simulink model "Proj2_P4"  (Simulink 8.6)
settings: Solver=ode45  StartTime=0.0  StopTime=10  MaxStep=0.001  RelTol=1e-3
values from neighbouring files (symbols this model uses):
  fl_rd_0 = fl_rd_rated    [Proj2_IM_IC_rated.m]    (also in Proj2_P1_calc.m = eps)
  fl_rd_0_est2 = fl_rd_rated_est2    [Proj2_P4_S2.m]    (also in Proj2_P4_calc2.m = fl_rd_0; Proj2_P4_calc3.m = fl_rd_0)
  fl_rd_0_est3 = fl_rd_rated    [Proj2_P4_S3.m]    (also in Proj2_P4_calc2.m = fl_rd_0; Proj2_P4_calc3.m = fl_rd_0)
  fl_sd_0 = fl_sd_rated    [Proj2_IM_IC_rated.m]    (also in Proj2_P1_calc.m = 0)
  fl_sq_0 = fl_sq_rated    [Proj2_IM_IC_rated.m]    (also in Proj2_P1_calc.m = 0)
  Isd_rated = real(Is_rated)    [Proj2_IM_IC_rated.m]
  Isd_rated_est2 = real(Is_rated_est2)    [Proj2_P4_S2.m]    (also in Proj2_P4_calc2.m = Isd_rated)
  Isd_rated_est3 = real(Is_rated_est3)    [Proj2_P4_S3.m]    (also in Proj2_P4_calc2.m = Isd_rated)
  Isq_0 = Isq_rated    [Proj2_IM_IC_rated.m]
  Isq_0_est2 = Isq_rated_est2    [Proj2_P4_S2.m]    (also in Proj2_P4_calc2.m = Isq_0; Proj2_P4_calc3.m = Isq_0)
  Isq_0_est3 = Isq_rated_est3    [Proj2_P4_S3.m]    (also in Proj2_P4_calc2.m = Isq_0; Proj2_P4_calc3.m = Isq_0)
  J_eq = 75    [Proj2_IM_parameters.m]
  Ki_i = w_c_i*sqrt(R_s^2+(w_c_i*L_s*sigma)^2) / sqrt(1+wc_Kp_by_Ki_for_i^2)    [Proj2_IM_IC_rated.m]
  Ki_i_est3 = w_c_i*sqrt(R_s^2+(w_c_i*L_s*sigma_est3)^2) / sqrt(1+wc_Kp_by_Ki_for_i_est3^2)    [Proj2_P4_S3.m]    (also in Proj2_P4_calc2.m = Ki_i)
  Ki_s = w_c_s^2*J_eq/(k*sqrt(1+tan(PM_s)^2))    [Proj2_IM_IC_rated.m]
  Ki_s_est2 = w_c_s^2*J_eq/(k_est2*sqrt(1+tan(PM_s)^2))    [Proj2_P4_S2.m]    (also in Proj2_P4_calc2.m = Ki_s)
  Ki_s_est3 = w_c_s^2*J_eq/(k_est3*sqrt(1+tan(PM_s)^2))    [Proj2_P4_S3.m]    (also in Proj2_P4_calc2.m = Ki_s)
  Kp_i = Ki_i * wc_Kp_by_Ki_for_i / w_c_i    [Proj2_IM_IC_rated.m]
  Kp_i_est3 = Ki_i_est3 * wc_Kp_by_Ki_for_i_est3 / w_c_i    [Proj2_P4_S3.m]    (also in Proj2_P4_calc2.m = Kp_i)
  Kp_s = Ki_s * wc_Kp_by_Ki_for_s / w_c_s    [Proj2_IM_IC_rated.m]
  Kp_s_est2 = Ki_s_est2 * wc_Kp_by_Ki_for_s / w_c_s    [Proj2_P4_S2.m]    (also in Proj2_P4_calc2.m = Kp_s)
  Kp_s_est3 = Ki_s_est3 * wc_Kp_by_Ki_for_s / w_c_s    [Proj2_P4_S3.m]    (also in Proj2_P4_calc2.m = Kp_s)
  L_m = X_m /w_syn    (= 0.00152788745368)    [Proj2_IM_parameters.m]
  L_r = L_lr+L_m    (= 0.00161011750761)    [Proj2_IM_parameters.m]
  L_r_est3 = L_lr_est3 + L_m    [Proj2_P4_S3.m]
  L_s = L_ls+L_m    (= 0.00161807525477)    [Proj2_IM_parameters.m]
  p = 6    [Proj2_IM_parameters.m]
  R_s = 1.4*10^-3    (= 0.0014)    [Proj2_IM_parameters.m]
  sigma = 1-L_m^2/(L_s*L_r)    (= 0.103961973695)    [Proj2_IM_parameters.m]
  sigma_est3 = 1-L_m^2/(L_s*L_r_est3)    [Proj2_P4_S3.m]
  T_L_rated = T_em_rated    [Proj2_IM_parameters.m]
  tau_r = L_r/R_r    (= 1.62474016914)    [Proj2_IM_parameters.m]
  tau_r_est2 = L_r/R_r_est2    [Proj2_P4_S2.m]
  tau_r_est3 = L_r_est3/R_r    [Proj2_P4_S3.m]
  theta_da_0 = theta_fl_rated_a    [Proj2_IM_IC_rated.m]    (also in Proj2_P1_calc.m = 0)
  theta_dA_0 = theta_fl_rated_a    [Proj2_IM_IC_rated.m]    (also in Proj2_P1_calc.m = 0)
  theta_da_0_est2 = theta_fl_rated_a_est2    [Proj2_P4_S2.m]    (also in Proj2_P4_calc2.m = theta_da_0; Proj2_P4_calc3.m = theta_da_0)
  theta_da_0_est3 = theta_fl_rated_a_est3    [Proj2_P4_S3.m]    (also in Proj2_P4_calc2.m = theta_da_0; Proj2_P4_calc3.m = theta_da_0)
  Vsd_prime_0 = Vsd_0 - L_m/L_r*d_fl_rd_0_by_dt + w_syn*sigma*L_s*Isq_0    [Proj2_IM_IC_rated.m]
  Vsd_prime_0_est2 = Vsd_0 - L_m/L_r*d_fl_rd_0_by_dt_est2 + w_syn*sigma*L_s*Isq_0_est2    [Proj2_P4_S2.m]    (also in Proj2_P4_calc2.m = Vsd_prime_0; Proj2_P4_calc3.m = Vsd_prime_0)
  Vsd_prime_0_est3 = Vsd_0 - L_m/L_r_est3*d_fl_rd_0_by_dt_est3 + w_syn*sigma_est3*L_s*Isq_0_est3    [Proj2_P4_S3.m]    (also in Proj2_P4_calc2.m = Vsd_prime_0; Proj2_P4_calc3.m = Vsd_prime_0)
  Vsq_prime_0 = Vsq_0 - w_syn*(L_m/L_r)*fl_rd_0 - w_syn*sigma*L_s*Isd_0    [Proj2_IM_IC_rated.m]
  Vsq_prime_0_est2 = Vsq_0 - w_syn*(L_m/L_r)*fl_rd_0_est2 - w_syn*sigma*L_s*Isd_0_est2    [Proj2_P4_S2.m]    (also in Proj2_P4_calc2.m = Vsq_prime_0; Proj2_P4_calc3.m = Vsq_prime_0)
  Vsq_prime_0_est3 = Vsq_0 - w_syn*(L_m/L_r_est3)*fl_rd_0_est3 - w_syn*sigma_est3*L_s*Isd_0_est3    [Proj2_P4_S3.m]    (also in Proj2_P4_calc2.m = Vsq_prime_0; Proj2_P4_calc3.m = Vsq_prime_0)
  w_mech_0 = w_mech_rated    [Proj2_IM_IC_rated.m]    (also in Proj2_P1_calc.m = 0)
  w_mech_rated = (1-s)*w_syn/(p/2)    (= 124.407069082)    [Proj2_IM_parameters.m]
(part 2 of 2)

== system Proj2_P4/Actual Motor dq Model Modified from EX5_3  /dq --> abc Eq. 2.10 ==
  d : Inport
  q : Inport  Port=2
  theta_da : Inport  Port=3
  Mux1 : Mux  Inputs=3
  ia Eq. 3-18 : Fcn  Expr=sqrt(2/3)*(cos(u(3))*u(1)-sin(u(3))*u(2))
  ib Eq. 3-18 : Fcn  Expr=sqrt(2/3)*(cos(u(3)+4*pi/3)*u(1)-sin(u(3)+4*pi/3)*u(2))
  ic Eq. 3-18 : Fcn  Expr=sqrt(2/3)*(cos(u(3)+2*pi/3)*u(1)-sin(u(3)+2*pi/3)*u(2))
  ia : Outport
  ib : Outport  Port=2
  ic : Outport  Port=3
  wires:
  ic Eq. 3-18/1 -> ic/1
  Mux1/1 -> ic Eq. 3-18/1, ib Eq. 3-18/1, ia Eq. 3-18/1
  ia Eq. 3-18/1 -> ia/1
  ib Eq. 3-18/1 -> ib/1
  d/1 -> Mux1/1
  q/1 -> Mux1/2
  theta_da/1 -> Mux1/3

== system Proj2_P4/Actual Motor dq Model Modified from EX5_3  /dq --> abc Eq. 2.16  ==
  d : Inport
  q : Inport  Port=2
  theta_dA : Inport  Port=3
  Mux1 : Mux  Inputs=3
  ia Eq. 3-18 : Fcn  Expr=sqrt(2/3)*(cos(u(3))*u(1)-sin(u(3))*u(2))
  ib Eq. 3-18 : Fcn  Expr=sqrt(2/3)*(cos(u(3)+4*pi/3)*u(1)-sin(u(3)+4*pi/3)*u(2))
  ic Eq. 3-18 : Fcn  Expr=sqrt(2/3)*(cos(u(3)+2*pi/3)*u(1)-sin(u(3)+2*pi/3)*u(2))
  i_A : Outport
  i_B : Outport  Port=2
  i_C : Outport  Port=3
  wires:
  ic Eq. 3-18/1 -> i_C/1
  Mux1/1 -> ic Eq. 3-18/1, ib Eq. 3-18/1, ia Eq. 3-18/1
  ib Eq. 3-18/1 -> i_B/1
  d/1 -> Mux1/1
  q/1 -> Mux1/2
  theta_dA/1 -> Mux1/3
  ia Eq. 3-18/1 -> i_A/1

== system Proj2_P4/Actual Motor dq Model Modified from EX5_3  /stator_flux Eq. 2.28 ==
  vs_dq : Inport
  is_dq : Inport  Port=2
  w_d : Inport  Port=3
  Gain : Gain  Gain=R_s  SaturateOnIntegerOverflow=on  OutDataTypeStr=Inherit: Same as input  ParamDataTypeStr=Inherit: Same as input
  Integrator1 : Integrator  InitialCondition=[fl_sd_0; fl_sq_0]
  "Matrix [0 -1  1 0] " : Gain  Gain=[0 -1; 1 0]  Multiplication=Matrix(K*u)  SaturateOnIntegerOverflow=on  OutDataTypeStr=Inherit: Same as input  ParamDataTypeStr=Inherit: Same as input
  Product : Product  SaturateOnIntegerOverflow=on  RndMeth=Zero  InputSameDT=on  OutDataTypeStr=Inherit: Same as first input
  Sum : Sum  Inputs=-+-  SaturateOnIntegerOverflow=on  InputSameDT=on  OutDataTypeStr=Inherit: Same as first input
  fl_s_dq : Outport
  wires:
  Sum/1 -> Integrator1/1
  Integrator1/1 -> "Matrix [0 -1  1 0] "/1, fl_s_dq/1
  "Matrix [0 -1  1 0] "/1 -> Product/2
  Product/1 -> Sum/1
  w_d/1 -> Product/1
  vs_dq/1 -> Sum/2
  is_dq/1 -> Gain/1
  Gain/1 -> Sum/3

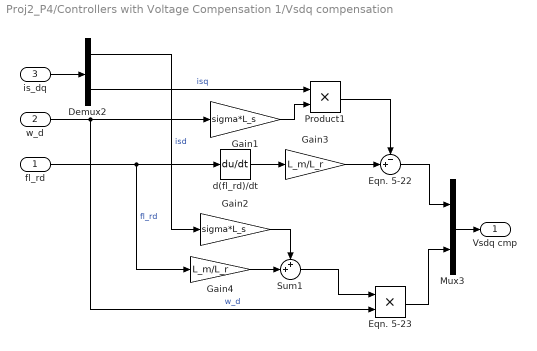
== system Proj2_P4/Controllers with Voltage Compensation 1/Vsdq compensation ==
  fl_rd : Inport
  w_d : Inport  Port=2
  is_dq : Inport  Port=3
  Demux2 : Demux  Outputs=2
  Eqn. 5-22 : Sum  Inputs=-+|  SaturateOnIntegerOverflow=on  InputSameDT=on  OutDataTypeStr=Inherit: Same as first input
  Eqn. 5-23 : Product  RndMeth=Zero
  Gain1 : Gain  Gain=sigma*L_s  SaturateOnIntegerOverflow=on  OutDataTypeStr=Inherit: Same as input  ParamDataTypeStr=Inherit: Same as input
  Gain2 : Gain  Gain=sigma*L_s  SaturateOnIntegerOverflow=on  OutDataTypeStr=Inherit: Same as input  ParamDataTypeStr=Inherit: Same as input
  Gain3 : Gain  Gain=L_m/L_r  SaturateOnIntegerOverflow=on  OutDataTypeStr=Inherit: Same as input  ParamDataTypeStr=Inherit: Same as input
  Gain4 : Gain  Gain=L_m/L_r  SaturateOnIntegerOverflow=on  OutDataTypeStr=Inherit: Same as input  ParamDataTypeStr=Inherit: Same as input
  Mux3 : Mux  Inputs=2
  Product1 : Product  RndMeth=Zero
  Sum1 : Sum  Inputs=++|  SaturateOnIntegerOverflow=on  InputSameDT=on  OutDataTypeStr=Inherit: Same as first input
  d(fl_rd)/dt : Derivative
  Vsdq cmp : Outport
  wires:
  fl_rd/1 -> d(fl_rd)/dt/1, Gain4/1  "fl_rd"
  d(fl_rd)/dt/1 -> Gain3/1
  Gain3/1 -> Eqn. 5-22/2
  w_d/1 -> Gain1/1, Eqn. 5-23/2  "w_d"
  Gain1/1 -> Product1/2
  Product1/1 -> Eqn. 5-22/1
  Eqn. 5-22/1 -> Mux3/1
  is_dq/1 -> Demux2/1
  Demux2/2 -> Product1/1  "isq"
  Gain4/1 -> Sum1/2
  Gain2/1 -> Sum1/1
  Sum1/1 -> Eqn. 5-23/1
  Eqn. 5-23/1 -> Mux3/2
  Demux2/1 -> Gain2/1  "isd"
  Mux3/1 -> Vsdq cmp/1

== system Proj2_P4/Controllers with Voltage Compensation 1/abc --> dq ==
  a : Inport
  b : Inport  Port=2
  c : Inport  Port=3
  theta_da_est : Inport  Port=4
  Mux1 : Mux
  isd Eq. 3-12 : Fcn  Expr=sqrt(2/3)*(cos(u(4))*u(1)+cos(u(4)-2*pi/3)*u(2)+cos(u(4)-4*pi/3)*u(3))
  isq Eq. 3-12 : Fcn  Expr=-sqrt(2/3)*(sin(u(4))*u(1)+sin(u(4)-2*pi/3)*u(2)+sin(u(4)-4*pi/3)*u(3))
  is_d : Outport
  is_q : Outport  Port=2
  wires:
  theta_da_est/1 -> Mux1/4
  c/1 -> Mux1/3
  b/1 -> Mux1/2
  a/1 -> Mux1/1
  isq Eq. 3-12/1 -> is_q/1
  isd Eq. 3-12/1 -> is_d/1
  Mux1/1 -> isq Eq. 3-12/1, isd Eq. 3-12/1

== system Proj2_P4/Controllers with Voltage Compensation 1/dq --> abc  ==
  d : Inport
  q : Inport  Port=2
  theta_da_est : Inport  Port=3
  Mux1 : Mux  Inputs=3
  ia Eq. 3-18 : Fcn  Expr=sqrt(2/3)*(cos(u(3))*u(1)-sin(u(3))*u(2))
  ib Eq. 3-18 : Fcn  Expr=sqrt(2/3)*(cos(u(3)+4*pi/3)*u(1)-sin(u(3)+4*pi/3)*u(2))
  ic Eq. 3-18 : Fcn  Expr=sqrt(2/3)*(cos(u(3)+2*pi/3)*u(1)-sin(u(3)+2*pi/3)*u(2))
  Va : Outport
  Vb : Outport  Port=2
  Vc : Outport  Port=3
  wires:
  ic Eq. 3-18/1 -> Vc/1
  Mux1/1 -> ic Eq. 3-18/1, ib Eq. 3-18/1, ia Eq. 3-18/1
  ib Eq. 3-18/1 -> Vb/1
  d/1 -> Mux1/1
  q/1 -> Mux1/2
  theta_da_est/1 -> Mux1/3
  ia Eq. 3-18/1 -> Va/1

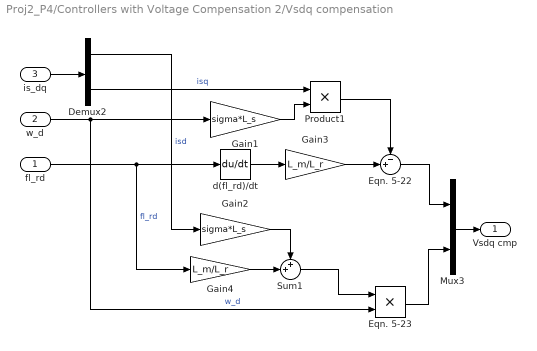
== system Proj2_P4/Controllers with Voltage Compensation 2/Vsdq compensation ==
  fl_rd : Inport
  w_d : Inport  Port=2
  is_dq : Inport  Port=3
  Demux2 : Demux  Outputs=2
  Eqn. 5-22 : Sum  Inputs=-+|  SaturateOnIntegerOverflow=on  InputSameDT=on  OutDataTypeStr=Inherit: Same as first input
  Eqn. 5-23 : Product  RndMeth=Zero
  Gain1 : Gain  Gain=sigma*L_s  SaturateOnIntegerOverflow=on  OutDataTypeStr=Inherit: Same as input  ParamDataTypeStr=Inherit: Same as input
  Gain2 : Gain  Gain=sigma*L_s  SaturateOnIntegerOverflow=on  OutDataTypeStr=Inherit: Same as input  ParamDataTypeStr=Inherit: Same as input
  Gain3 : Gain  Gain=L_m/L_r  SaturateOnIntegerOverflow=on  OutDataTypeStr=Inherit: Same as input  ParamDataTypeStr=Inherit: Same as input
  Gain4 : Gain  Gain=L_m/L_r  SaturateOnIntegerOverflow=on  OutDataTypeStr=Inherit: Same as input  ParamDataTypeStr=Inherit: Same as input
  Mux3 : Mux  Inputs=2
  Product1 : Product  RndMeth=Zero
  Sum1 : Sum  Inputs=++|  SaturateOnIntegerOverflow=on  InputSameDT=on  OutDataTypeStr=Inherit: Same as first input
  d(fl_rd)/dt : Derivative
  Vsdq cmp : Outport
  wires:
  fl_rd/1 -> d(fl_rd)/dt/1, Gain4/1  "fl_rd"
  d(fl_rd)/dt/1 -> Gain3/1
  Gain3/1 -> Eqn. 5-22/2
  w_d/1 -> Gain1/1, Eqn. 5-23/2  "w_d"
  Gain1/1 -> Product1/2
  Product1/1 -> Eqn. 5-22/1
  Eqn. 5-22/1 -> Mux3/1
  is_dq/1 -> Demux2/1
  Demux2/2 -> Product1/1  "isq"
  Gain4/1 -> Sum1/2
  Gain2/1 -> Sum1/1
  Sum1/1 -> Eqn. 5-23/1
  Eqn. 5-23/1 -> Mux3/2
  Demux2/1 -> Gain2/1  "isd"
  Mux3/1 -> Vsdq cmp/1

== system Proj2_P4/Controllers with Voltage Compensation 2/abc --> dq  ==
  a : Inport
  b : Inport  Port=2
  c : Inport  Port=3
  theta_da_est : Inport  Port=4
  Mux1 : Mux
  isd Eq. 3-12 : Fcn  Expr=sqrt(2/3)*(cos(u(4))*u(1)+cos(u(4)-2*pi/3)*u(2)+cos(u(4)-4*pi/3)*u(3))
  isq Eq. 3-12 : Fcn  Expr=-sqrt(2/3)*(sin(u(4))*u(1)+sin(u(4)-2*pi/3)*u(2)+sin(u(4)-4*pi/3)*u(3))
  is_d : Outport
  is_q : Outport  Port=2
  wires:
  theta_da_est/1 -> Mux1/4
  c/1 -> Mux1/3
  b/1 -> Mux1/2
  a/1 -> Mux1/1
  isq Eq. 3-12/1 -> is_q/1
  isd Eq. 3-12/1 -> is_d/1
  Mux1/1 -> isq Eq. 3-12/1, isd Eq. 3-12/1

== system Proj2_P4/Controllers with Voltage Compensation 2/dq --> abc  ==
  d : Inport
  q : Inport  Port=2
  theta_da_est : Inport  Port=3
  Mux1 : Mux  Inputs=3
  ia Eq. 3-18 : Fcn  Expr=sqrt(2/3)*(cos(u(3))*u(1)-sin(u(3))*u(2))
  ib Eq. 3-18 : Fcn  Expr=sqrt(2/3)*(cos(u(3)+4*pi/3)*u(1)-sin(u(3)+4*pi/3)*u(2))
  ic Eq. 3-18 : Fcn  Expr=sqrt(2/3)*(cos(u(3)+2*pi/3)*u(1)-sin(u(3)+2*pi/3)*u(2))
  Va : Outport
  Vb : Outport  Port=2
  Vc : Outport  Port=3
  wires:
  ic Eq. 3-18/1 -> Vc/1
  Mux1/1 -> ic Eq. 3-18/1, ib Eq. 3-18/1, ia Eq. 3-18/1
  ib Eq. 3-18/1 -> Vb/1
  d/1 -> Mux1/1
  q/1 -> Mux1/2
  theta_da_est/1 -> Mux1/3
  ia Eq. 3-18/1 -> Va/1

== system Proj2_P4/Controllers with Voltage Compensation 3/Vsdq compensation ==
  fl_rd : Inport
  w_d : Inport  Port=2
  is_dq : Inport  Port=3
  Demux2 : Demux  Outputs=2
  Eqn. 5-22 : Sum  Inputs=-+|  SaturateOnIntegerOverflow=on  InputSameDT=on  OutDataTypeStr=Inherit: Same as first input
  Eqn. 5-23 : Product  RndMeth=Zero
  Gain1 : Gain  Gain=sigma_est3*L_s  SaturateOnIntegerOverflow=on  OutDataTypeStr=Inherit: Same as input  ParamDataTypeStr=Inherit: Same as input
  Gain2 : Gain  Gain=sigma_est3*L_s  SaturateOnIntegerOverflow=on  OutDataTypeStr=Inherit: Same as input  ParamDataTypeStr=Inherit: Same as input
  Gain3 : Gain  Gain=L_m/L_r_est3  SaturateOnIntegerOverflow=on  OutDataTypeStr=Inherit: Same as input  ParamDataTypeStr=Inherit: Same as input
  Gain4 : Gain  Gain=L_m/L_r_est3  SaturateOnIntegerOverflow=on  OutDataTypeStr=Inherit: Same as input  ParamDataTypeStr=Inherit: Same as input
  Mux3 : Mux  Inputs=2
  Product1 : Product  RndMeth=Zero
  Sum1 : Sum  Inputs=++|  SaturateOnIntegerOverflow=on  InputSameDT=on  OutDataTypeStr=Inherit: Same as first input
  d(fl_rd)/dt : Derivative
  Vsdq cmp : Outport
  wires:
  fl_rd/1 -> d(fl_rd)/dt/1, Gain4/1  "fl_rd"
  d(fl_rd)/dt/1 -> Gain3/1
  Gain3/1 -> Eqn. 5-22/2
  w_d/1 -> Gain1/1, Eqn. 5-23/2  "w_d"
  Gain1/1 -> Product1/2
  Product1/1 -> Eqn. 5-22/1
  Eqn. 5-22/1 -> Mux3/1
  is_dq/1 -> Demux2/1
  Demux2/2 -> Product1/1  "isq"
  Gain4/1 -> Sum1/2
  Gain2/1 -> Sum1/1
  Sum1/1 -> Eqn. 5-23/1
  Eqn. 5-23/1 -> Mux3/2
  Demux2/1 -> Gain2/1  "isd"
  Mux3/1 -> Vsdq cmp/1

== system Proj2_P4/Controllers with Voltage Compensation 3/abc --> dq  ==
  a : Inport
  b : Inport  Port=2
  c : Inport  Port=3
  theta_da_est : Inport  Port=4
  Mux1 : Mux
  isd Eq. 3-12 : Fcn  Expr=sqrt(2/3)*(cos(u(4))*u(1)+cos(u(4)-2*pi/3)*u(2)+cos(u(4)-4*pi/3)*u(3))
  isq Eq. 3-12 : Fcn  Expr=-sqrt(2/3)*(sin(u(4))*u(1)+sin(u(4)-2*pi/3)*u(2)+sin(u(4)-4*pi/3)*u(3))
  is_d : Outport
  is_q : Outport  Port=2
  wires:
  theta_da_est/1 -> Mux1/4
  c/1 -> Mux1/3
  b/1 -> Mux1/2
  a/1 -> Mux1/1
  isq Eq. 3-12/1 -> is_q/1
  isd Eq. 3-12/1 -> is_d/1
  Mux1/1 -> isq Eq. 3-12/1, isd Eq. 3-12/1

== system Proj2_P4/Controllers with Voltage Compensation 3/dq --> abc  ==
  d : Inport
  q : Inport  Port=2
  theta_da_est : Inport  Port=3
  Mux1 : Mux  Inputs=3
  ia Eq. 3-18 : Fcn  Expr=sqrt(2/3)*(cos(u(3))*u(1)-sin(u(3))*u(2))
  ib Eq. 3-18 : Fcn  Expr=sqrt(2/3)*(cos(u(3)+4*pi/3)*u(1)-sin(u(3)+4*pi/3)*u(2))
  ic Eq. 3-18 : Fcn  Expr=sqrt(2/3)*(cos(u(3)+2*pi/3)*u(1)-sin(u(3)+2*pi/3)*u(2))
  Va : Outport
  Vb : Outport  Port=2
  Vc : Outport  Port=3
  wires:
  ic Eq. 3-18/1 -> Vc/1
  Mux1/1 -> ic Eq. 3-18/1, ib Eq. 3-18/1, ia Eq. 3-18/1
  ib Eq. 3-18/1 -> Vb/1
  d/1 -> Mux1/1
  q/1 -> Mux1/2
  theta_da_est/1 -> Mux1/3
  ia Eq. 3-18/1 -> Va/1

== system Proj2_P4/Estimated Motor Model/abc --> dq Eq. 3-12 ==
  a : Inport
  b : Inport  Port=2
  c : Inport  Port=3
  theta_da_est : Inport  Port=4
  Mux1 : Mux
  Mux2 : Mux  Inputs=2
  isd Eq. 3-8 : Fcn  Expr=sqrt(2/3)*(cos(u(4))*u(1)+cos(u(4)-2*pi/3)*u(2)+cos(u(4)-4*pi/3)*u(3))
  vsq Eq. 3-8 : Fcn  Expr=-sqrt(2/3)*(sin(u(4))*u(1)+sin(u(4)-2*pi/3)*u(2)+sin(u(4)-4*pi/3)*u(3))
  is_dq : Outport
  wires:
  Mux2/1 -> is_dq/1
  theta_da_est/1 -> Mux1/4
  c/1 -> Mux1/3
  b/1 -> Mux1/2
  a/1 -> Mux1/1
  vsq Eq. 3-8/1 -> Mux2/2
  isd Eq. 3-8/1 -> Mux2/1
  Mux1/1 -> vsq Eq. 3-8/1, isd Eq. 3-8/1

== system Proj2_P4/Estimated Motor Model 2/abc --> dq Eq. 3-12 ==
  a : Inport
  b : Inport  Port=2
  c : Inport  Port=3
  theta_da_est : Inport  Port=4
  Mux1 : Mux
  Mux2 : Mux  Inputs=2
  isd Eq. 3-8 : Fcn  Expr=sqrt(2/3)*(cos(u(4))*u(1)+cos(u(4)-2*pi/3)*u(2)+cos(u(4)-4*pi/3)*u(3))
  vsq Eq. 3-8 : Fcn  Expr=-sqrt(2/3)*(sin(u(4))*u(1)+sin(u(4)-2*pi/3)*u(2)+sin(u(4)-4*pi/3)*u(3))
  is_dq : Outport
  wires:
  Mux2/1 -> is_dq/1
  theta_da_est/1 -> Mux1/4
  c/1 -> Mux1/3
  b/1 -> Mux1/2
  a/1 -> Mux1/1
  vsq Eq. 3-8/1 -> Mux2/2
  isd Eq. 3-8/1 -> Mux2/1
  Mux1/1 -> vsq Eq. 3-8/1, isd Eq. 3-8/1

== system Proj2_P4/Estimated Motor Model 3/abc --> dq Eq. 3-12 ==
  a : Inport
  b : Inport  Port=2
  c : Inport  Port=3
  theta_da_est : Inport  Port=4
  Mux1 : Mux
  Mux2 : Mux  Inputs=2
  isd Eq. 3-8 : Fcn  Expr=sqrt(2/3)*(cos(u(4))*u(1)+cos(u(4)-2*pi/3)*u(2)+cos(u(4)-4*pi/3)*u(3))
  vsq Eq. 3-8 : Fcn  Expr=-sqrt(2/3)*(sin(u(4))*u(1)+sin(u(4)-2*pi/3)*u(2)+sin(u(4)-4*pi/3)*u(3))
  is_dq : Outport
  wires:
  Mux2/1 -> is_dq/1
  theta_da_est/1 -> Mux1/4
  c/1 -> Mux1/3
  b/1 -> Mux1/2
  a/1 -> Mux1/1
  vsq Eq. 3-8/1 -> Mux2/2
  isd Eq. 3-8/1 -> Mux2/1
  Mux1/1 -> vsq Eq. 3-8/1, isd Eq. 3-8/1
